simulink model "Seat_PC_Model"  (R2020a)
settings: Solver=FixedStepDiscrete  StartTime=0.0  StopTime=50  FixedStep=1  RelTol=1e-3
undefined symbols (not defined in the file or in its folder): Seat_PC_System
libraries: simulink x1
settings Model: Creator=A  LastModifiedBy=A

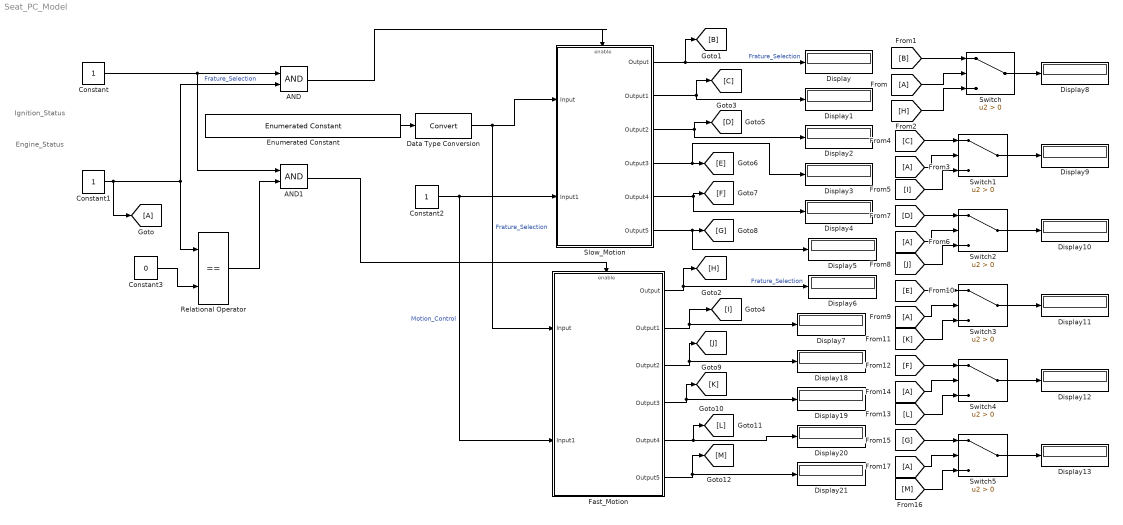
== system Seat_PC_Model ==
  note: Engine_Status
  note: Ignition_Status
  AND : Logic  AllPortsSameDT=off  OutDataTypeStr=boolean
  AND1 : Logic  AllPortsSameDT=off  OutDataTypeStr=boolean
  Constant : Constant
  Constant1 : Constant
  Constant2 : Constant
  Constant3 : Constant  Value=0
  Data Type Conversion : DataTypeConversion
  Display{,1..13,18..21} (18 alike) : Display
  Enumerated Constant : simulink/Sources/Enumerated Constant  OutDataTypeStr=Enum:Seat_PC_System  Value=Seat_PC_System.Forward_Backward_M  SampleTime=inf
  Fast_Motion : Subsystem
  Relational Operator : RelationalOperator  Operator===  OutDataTypeStr=boolean  RndMeth=Simplest
  Slow_Motion : Subsystem
  Switch{,1..5} (6 alike) : Switch  Criteria=u2 > Threshold
  wires:
  AND/1 -> Slow_Motion/Enable
  AND1/1 -> Fast_Motion/Enable
  Constant/1 -> AND1/1, AND/1
  Constant3/1 -> Relational Operator/2
  Relational Operator/1 -> AND1/2
  Slow_Motion/2(Output1) -> Display1/1, [C]
  Slow_Motion/3(Output2) -> Display2/1, [D]
  Slow_Motion/4(Output3) -> Display3/1, [E]
  Slow_Motion/5(Output4) -> Display4/1, [F]
  Slow_Motion/6(Output5) -> Display5/1, [G]
  Fast_Motion/6(Output5) -> [M], Display21/1
  Fast_Motion/4(Output3) -> [K], Display19/1
  Fast_Motion/5(Output4) -> [L], Display20/1
  Fast_Motion/3(Output2) -> [J], Display18/1
  Fast_Motion/2(Output1) -> [I], Display7/1
  Fast_Motion/1(Output) -> [H], Display6/1  "Frature_Selection"
  Slow_Motion/1(Output) -> Display/1, [B]  "Frature_Selection"
  Switch/1 -> Display8/1
  [A] -> Switch/2
  [B] -> Switch/1
  [H] -> Switch/3
  [I] -> Switch1/3
  [C] -> Switch1/1
  [A] -> Switch1/2
  Switch1/1 -> Display9/1
  Switch2/1 -> Display10/1
  [A] -> Switch2/2
  [D] -> Switch2/1
  [J] -> Switch2/3
  [K] -> Switch3/3
  [E] -> Switch3/1
  [A] -> Switch3/2
  Switch3/1 -> Display11/1
  Switch4/1 -> Display12/1
  [A] -> Switch4/2
  [F] -> Switch4/1
  [L] -> Switch4/3
  [M] -> Switch5/3
  [G] -> Switch5/1
  [A] -> Switch5/2
  Switch5/1 -> Display13/1
  Constant1/1 -> AND/2, Relational Operator/1, [A]  "Frature_Selection"
  Enumerated Constant/1 -> Data Type Conversion/1
  Constant2/1 -> Fast_Motion/2(Input1), Slow_Motion/2(Input1)  "Motion_Control"
  Data Type Conversion/1 -> Fast_Motion/1(Input), Slow_Motion/1(Input)  "Frature_Selection"

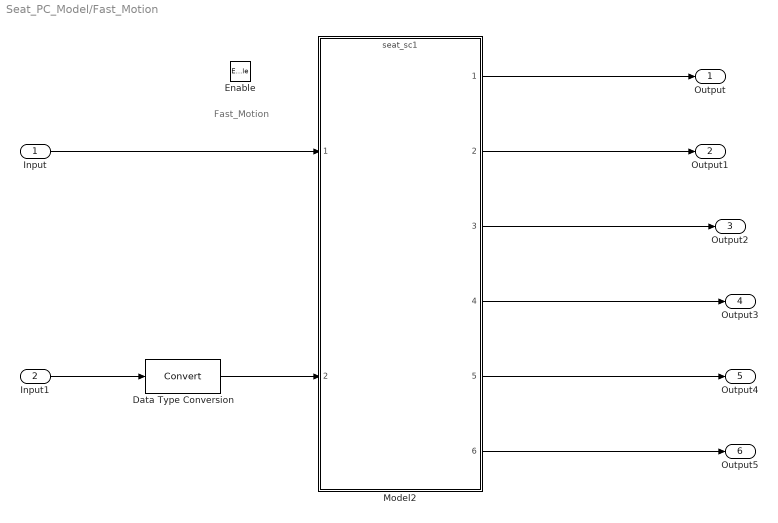
== system Seat_PC_Model/Fast_Motion ==
  note: Fast_Motion
  Input : Inport
  Input1 : Inport  Port=2
  Enable : EnablePort
  Data Type Conversion : DataTypeConversion
  Model2 : ModelReference  ModelNameDialog=seat_sc1.slx  SimulationMode=Normal  ModelReferenceVersion=1.19
  Output : Outport
  Output1 : Outport  Port=2
  Output2 : Outport  Port=3
  Output3 : Outport  Port=4
  Output4 : Outport  Port=5
  Output5 : Outport  Port=6
  wires:
  Model2/1 -> Output/1
  Model2/2 -> Output1/1
  Model2/3 -> Output2/1
  Model2/4 -> Output3/1
  Model2/5 -> Output4/1
  Model2/6 -> Output5/1
  Input/1 -> Model2/1
  Input1/1 -> Data Type Conversion/1
  Data Type Conversion/1 -> Model2/2

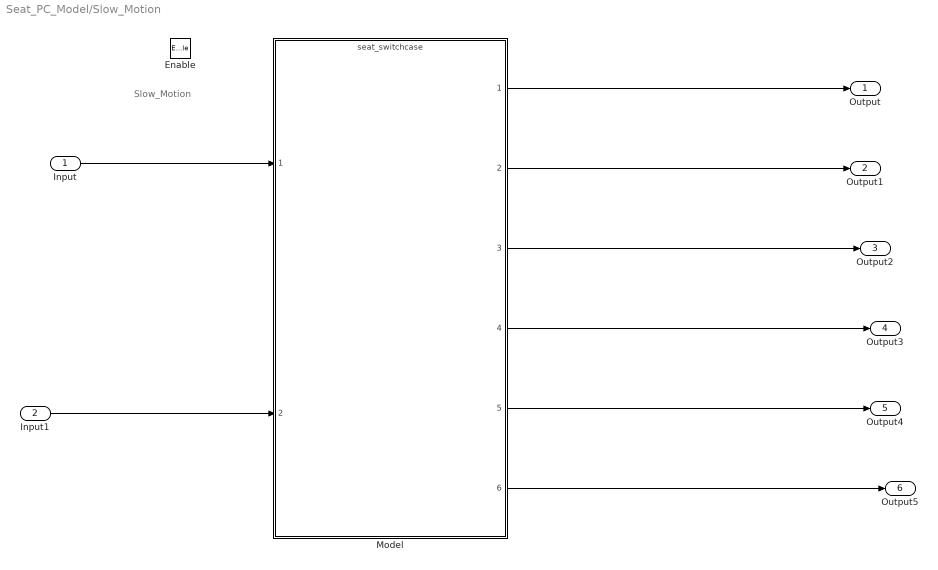
== system Seat_PC_Model/Slow_Motion ==
  note: Slow_Motion
  Input : Inport
  Input1 : Inport  Port=2
  Enable : EnablePort
  Model : ModelReference  ModelNameDialog=seat_switchcase.slx  SimulationMode=Normal  ModelReferenceVersion=1.35
  Output : Outport
  Output1 : Outport  Port=2
  Output2 : Outport  Port=3
  Output3 : Outport  Port=4
  Output4 : Outport  Port=5
  Output5 : Outport  Port=6
  wires:
  Model/2 -> Output1/1
  Model/1 -> Output/1
  Model/3 -> Output2/1
  Model/4 -> Output3/1
  Model/5 -> Output4/1
  Model/6 -> Output5/1
  Input/1 -> Model/1
  Input1/1 -> Model/2
